simulink model "tesr"  (R2021a)
settings: Solver=VariableStepAuto  StartTime=0.0  StopTime=10.0  RelTol=1e-3
libraries: commchan3 x1, dsparch4 x1
settings Model: Creator=Safir  LastModifiedBy=Safir

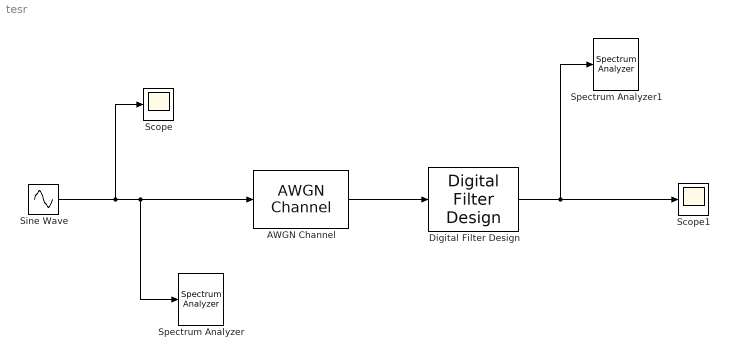
== system tesr ==
  AWGN Channel : commchan3/AWGN Channel  InputProcessing=Columns as channels (frame based)  seed=67  noiseMode="Signal to noise ratio  (Eb/No)"  EbNodB=10  EsNodB=10  SNRdB=10  bitsPerSym=1  Ps=1  Tsym=1  variance=1
  Digital Filter Design : dsparch4/Digital Filter Design  mwdsp_browser_bugfix_var=off
  Scope : Scope
  Scope1 : Scope
  Sine Wave : Sin  SampleTime=0
  Spectrum Analyzer : SpectrumAnalyzer
  Spectrum Analyzer1 : SpectrumAnalyzer
  wires:
  Sine Wave/1 -> Scope/1, Spectrum Analyzer/1, AWGN Channel/1
  AWGN Channel/1 -> Digital Filter Design/1
  Digital Filter Design/1 -> Spectrum Analyzer1/1, Scope1/1
